simulink model "elastic_robot_arm_robust_controller"  (R2018b)
settings: Solver=ode8  StartTime=0.0  StopTime=50  FixedStep=0.001  RelTol=1e-3
undefined symbols (not defined in the file or in its folder): sigbuilder_block
settings Model: Creator=TUAN HUA  LastModifiedBy=Tuan Hua

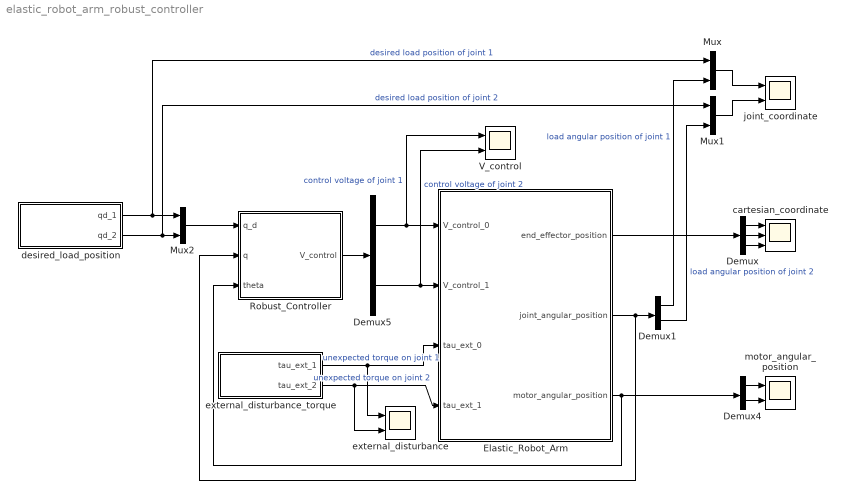
== system elastic_robot_arm_robust_controller ==
  Demux : Demux  Outputs=3
  Demux1 : Demux  Outputs=2
  Demux4 : Demux  Outputs=2
  Demux5 : Demux  Outputs=2
  Elastic_Robot_Arm : Subsystem  mask{ml0=6, Ilzz0=0.1, K0=1200.0, ml1=4, Ilzz1=0.1, K1=1440.0}
      mask prompts: ml0 "Link mass (kg) (defaut: 6)"; Ilzz0 "Link inertia (kg·m^2) (defaut: 0.1)"; K0 "Spring stiffness (N/m) (default: 1500)"; ml1 "Link mass (kg) (defaut: 4)"; Ilzz1 "Link inertia (kg·m^2) (defaut: 0.1)"; K1 "Spring stiffness (N/m) (default: 1200)"
      mask DialogControl Container1 Prompt: Joint 1
      mask DialogControl Container2 Prompt: Joint 2
      mask DialogControl Control1 Prompt: Reset to default
      mask DialogControl Control1 Callback:
      | robot_model = Simulink.Mask.get('elastic_robot_arm_robust_controller/Elastic_Robot_Arm');
      | 
      | % ml0
      | param = robot_model.Parameters(1);
      | param.set('Value', '6');
      | 
      | % Ilzz0
      | param = robot_model.Parameters(2);
      | param.set('Value', '0.1');
      | 
      | % K0
      | param = robot_model.Parameters(3);
      | param.set('Value', '1500');
      | 
      | % ml1
      | param = robot_model.Parameters(4);
      | param.set('Value', '4');
      | 
      | % Ilzz1
      | param = robot_model.Parameters(5);
      | param.set('Value', '0.1');
      | 
      | % K1
      | param = robot_model.Parameters(6);
      | param.set('Value', '1200');
  Mux : Mux  Inputs=2
  Mux1 : Mux  Inputs=2
  Mux2 : Mux  Inputs=2
  Robust_Controller : Subsystem
  V_control : Scope  NumInputPorts=2
  cartesian_coordinate : Scope  NumInputPorts=3
  desired_load_position : Subsystem  mask{inputType=Sine Waveform Input}
      mask prompts: inputType "Input Type"
      mask TypeOptions inputType: Sine Waveform Input | Square Waveform Input | Arbitrary Waveform Input
  external_disturbance : Scope  NumInputPorts=2
  external_disturbance_torque : Subsystem  mask{unexpectedTorqueType=No External Disturbance}
      mask prompts: unexpectedTorqueType "Unexpected Torque Type"
      mask TypeOptions unexpectedTorqueType: No External Disturbance | Unexpected Torque In Sine Waveform | Unexpected Torque In Pulse Form
  joint_coordinate : Scope  NumInputPorts=2
  motor_angular_position : Scope  NumInputPorts=2
  wires:
  Demux/3 -> cartesian_coordinate/3
  Demux/2 -> cartesian_coordinate/2
  Demux/1 -> cartesian_coordinate/1
  Elastic_Robot_Arm/1(end_effector_position) -> Demux/1
  Elastic_Robot_Arm/2(joint_angular_position) -> Robust_Controller/2(q), Demux1/1
  Elastic_Robot_Arm/3(motor_angular_position) -> Robust_Controller/3(theta), Demux4/1
  desired_load_position/1(qd_1) -> Mux/1, Mux2/1  "desired load position of joint 1"
  desired_load_position/2(qd_2) -> Mux1/1, Mux2/2  "desired load position of joint 2"
  Demux4/1 -> motor_angular_position/1
  Demux4/2 -> motor_angular_position/2
  Demux1/1 -> Mux/2  "load angular position of joint 1"
  Demux1/2 -> Mux1/2  "load angular position of joint 2"
  Mux/1 -> joint_coordinate/1
  Mux1/1 -> joint_coordinate/2
  Robust_Controller/1(V_control) -> Demux5/1
  Demux5/2 -> Elastic_Robot_Arm/2(V_control_1), V_control/2  "control voltage of joint 2"
  Demux5/1 -> Elastic_Robot_Arm/1(V_control_0), V_control/1  "control voltage of joint 1"
  Mux2/1 -> Robust_Controller/1(q_d)
  external_disturbance_torque/1(tau_ext_1) -> Elastic_Robot_Arm/3(tau_ext_0), external_disturbance/1  "unexpected torque on joint 1"
  external_disturbance_torque/2(tau_ext_2) -> Elastic_Robot_Arm/4(tau_ext_1), external_disturbance/2  "unexpected torque on joint 2"

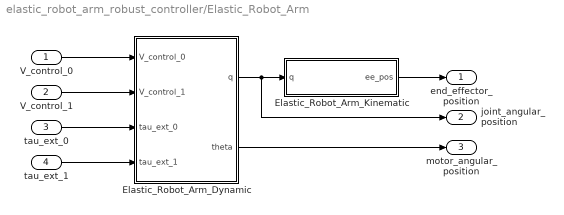
== system elastic_robot_arm_robust_controller/Elastic_Robot_Arm ==
  V_control_0 : Inport
  V_control_1 : Inport  Port=2
  tau_ext_0 : Inport  Port=3
  tau_ext_1 : Inport  Port=4
  Elastic_Robot_Arm_Dynamic : Subsystem
  Elastic_Robot_Arm_Kinematic : Subsystem
  end_effector_position : Outport
  joint_angular_position : Outport  Port=2
  motor_angular_position : Outport  Port=3
  wires:
  Elastic_Robot_Arm_Dynamic/2(theta) -> motor_angular_position/1
  Elastic_Robot_Arm_Kinematic/1(ee_pos) -> end_effector_position/1
  tau_ext_1/1 -> Elastic_Robot_Arm_Dynamic/4(tau_ext_1)
  tau_ext_0/1 -> Elastic_Robot_Arm_Dynamic/3(tau_ext_0)
  V_control_1/1 -> Elastic_Robot_Arm_Dynamic/2(V_control_1)
  V_control_0/1 -> Elastic_Robot_Arm_Dynamic/1(V_control_0)
  Elastic_Robot_Arm_Dynamic/1(q) -> Elastic_Robot_Arm_Kinematic/1(q), joint_angular_position/1

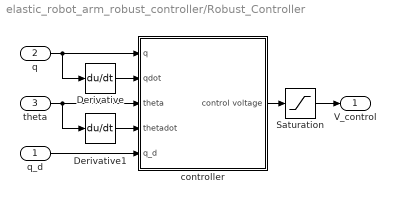
== system elastic_robot_arm_robust_controller/Robust_Controller ==
  q_d : Inport
  q : Inport  Port=2
  theta : Inport  Port=3
  Derivative : Derivative  CoefficientInTFapproximation=0
  Derivative1 : Derivative  CoefficientInTFapproximation=0
  Saturation : Saturate  UpperLimit=12  LowerLimit=-12
  controller : Subsystem
  V_control : Outport
  wires:
  q/1 -> controller/1(q), Derivative/1
  Derivative/1 -> controller/2(qdot)
  theta/1 -> Derivative1/1, controller/3(theta)
  Derivative1/1 -> controller/4(thetadot)
  q_d/1 -> controller/5(q_d)
  controller/1(control voltage) -> Saturation/1
  Saturation/1 -> V_control/1

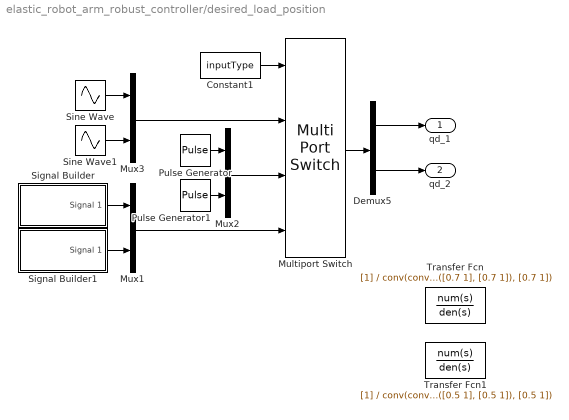
== system elastic_robot_arm_robust_controller/desired_load_position ==
  Constant1 : Constant  Value=inputType  OutDataTypeStr=uint8
  Demux5 : Demux  Outputs=2
  Multiport Switch : MultiPortSwitch
  Mux1 : Mux  Inputs=2
  Mux2 : Mux  Inputs=2
  Mux3 : Mux  Inputs=2
  Pulse Generator : DiscretePulseGenerator  PulseType=Time based  Period=20  PulseWidth=50
  Pulse Generator1 : DiscretePulseGenerator  PulseType=Time based  Period=20  PulseWidth=50
  Signal Builder : Subsystem  Tag=STV Subsys  LoadFcn=sigbuilder_block('load');  StartFcn=sigbuilder_block('start');  StopFcn=sigbuilder_block('stop');  ClipboardFcn=sigbuilder_block('clipboard');  mask(Sigbuilder block){tuvar=[0:10]}
      mask help: Simulink:masks:SigbuilderBlock_MD
      mask init:
      | if ~strcmp(get_param(bdroot(gcbh),'SimulationStatus'),'stopped') tuvar = sigbuilder_block('maskInit'); end
      settings: CopyFcn=sigbuilder_block('copy');  DeleteFcn=sigbuilder_block('delete');  ModelCloseFcn=sigbuilder_block('modelClose');  PreSaveFcn=sigbuilder_block('preSave');  PauseFcn=sigbuilder_block('pause');  ContinueFcn=sigbuilder_block('continue');  NameChangeFcn=sigbuilder_block('namechange');  OpenFcn=sigbuilder_block('open',[6 3 1012.5 474 ]);  CloseFcn=sigbuilder_block('close');
      mask Display: plot(0, 0, 100, 100,[2, 2, 32, 32, 2], [68, 8, 8, 68, 68],[32, 2], [38, 38], [32, 19, 2],[53, 60, 44], [32, 17, 17, 2],[16, 16, 31, 31]);txt = getActiveGroup(gcbh);text(2, 100, txt,'verticalAlignment', 'top');
  Signal Builder1 : Subsystem  Tag=STV Subsys  LoadFcn=sigbuilder_block('load');  StartFcn=sigbuilder_block('start');  StopFcn=sigbuilder_block('stop');  ClipboardFcn=sigbuilder_block('clipboard');  mask(Sigbuilder block){tuvar=[0:10]}
      mask help: Simulink:masks:SigbuilderBlock_MD
      mask init:
      | if ~strcmp(get_param(bdroot(gcbh),'SimulationStatus'),'stopped') tuvar = sigbuilder_block('maskInit'); end
      settings: CopyFcn=sigbuilder_block('copy');  DeleteFcn=sigbuilder_block('delete');  ModelCloseFcn=sigbuilder_block('modelClose');  PreSaveFcn=sigbuilder_block('preSave');  PauseFcn=sigbuilder_block('pause');  ContinueFcn=sigbuilder_block('continue');  NameChangeFcn=sigbuilder_block('namechange');  OpenFcn=sigbuilder_block('open',[6 0 1012.5 477.75 ]);  CloseFcn=sigbuilder_block('close');
      mask Display: plot(0, 0, 100, 100,[2, 2, 32, 32, 2], [68, 8, 8, 68, 68],[32, 2], [38, 38], [32, 19, 2],[53, 60, 44], [32, 17, 17, 2],[16, 16, 31, 31]);txt = getActiveGroup(gcbh);text(2, 100, txt,'verticalAlignment', 'top');
  Sine Wave : Sin  Frequency=0.25*pi  SampleTime=0
  Sine Wave1 : Sin  Frequency=0.25*pi  SampleTime=0
  Transfer Fcn : TransferFcn  Denominator=conv(conv([0.7 1], [0.7 1]), [0.7 1])
  Transfer Fcn1 : TransferFcn  Denominator=conv(conv([0.5 1], [0.5 1]), [0.5 1])
  qd_1 : Outport
  qd_2 : Outport  Port=2
  wires:
  Mux1/1 -> Multiport Switch/4
  Signal Builder1/1(Signal 1) -> Mux1/2
  Signal Builder/1(Signal 1) -> Mux1/1
  Demux5/2 -> qd_2/1
  Demux5/1 -> qd_1/1
  Constant1/1 -> Multiport Switch/1
  Sine Wave1/1 -> Mux3/2
  Mux2/1 -> Multiport Switch/3
  Pulse Generator/1 -> Mux2/1
  Pulse Generator1/1 -> Mux2/2
  Multiport Switch/1 -> Demux5/1
  Sine Wave/1 -> Mux3/1
  Mux3/1 -> Multiport Switch/2

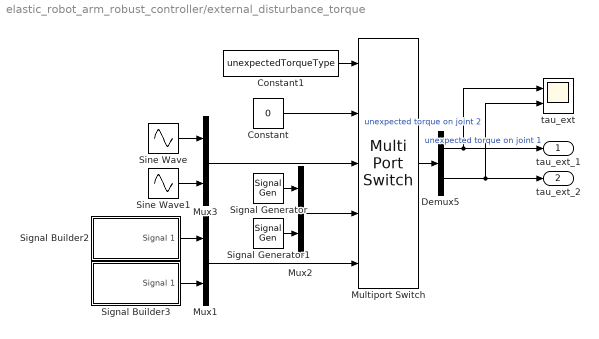
== system elastic_robot_arm_robust_controller/external_disturbance_torque ==
  Constant : Constant  Value=0
  Constant1 : Constant  Value=unexpectedTorqueType  OutDataTypeStr=uint8
  Demux5 : Demux  Outputs=2
  Multiport Switch : MultiPortSwitch  Inputs=4
  Mux1 : Mux  Inputs=2
  Mux2 : Mux  Inputs=2
  Mux3 : Mux  Inputs=2
  Signal Generator : SignalGenerator  WaveForm=square  Frequency=pi  Units=rad/sec
  Signal Generator1 : SignalGenerator  WaveForm=square  Frequency=0.5*pi  Units=rad/sec
  Signal Builder2 : Subsystem  Tag=STV Subsys  LoadFcn=sigbuilder_block('load');  StartFcn=sigbuilder_block('start');  StopFcn=sigbuilder_block('stop');  ClipboardFcn=sigbuilder_block('clipboard');  mask(Sigbuilder block){tuvar=[0:10]}
      mask help: Simulink:masks:SigbuilderBlock_MD
      mask init:
      | if ~strcmp(get_param(bdroot(gcbh),'SimulationStatus'),'stopped') tuvar = sigbuilder_block('maskInit'); end
      settings: CopyFcn=sigbuilder_block('copy');  DeleteFcn=sigbuilder_block('delete');  ModelCloseFcn=sigbuilder_block('modelClose');  PreSaveFcn=sigbuilder_block('preSave');  PauseFcn=sigbuilder_block('pause');  ContinueFcn=sigbuilder_block('continue');  NameChangeFcn=sigbuilder_block('namechange');  OpenFcn=sigbuilder_block('open',[0.75 27 1006.5 433.5 ]);  CloseFcn=sigbuilder_block('close');
      mask Display: plot(0, 0, 100, 100,[2, 2, 32, 32, 2], [68, 8, 8, 68, 68],[32, 2], [38, 38], [32, 19, 2],[53, 60, 44], [32, 17, 17, 2],[16, 16, 31, 31]);txt = getActiveGroup(gcbh);text(2, 100, txt,'verticalAlignment', 'top');
  Signal Builder3 : Subsystem  Tag=STV Subsys  LoadFcn=sigbuilder_block('load');  StartFcn=sigbuilder_block('start');  StopFcn=sigbuilder_block('stop');  ClipboardFcn=sigbuilder_block('clipboard');  mask(Sigbuilder block){tuvar=[0:10]}
      mask help: Simulink:masks:SigbuilderBlock_MD
      mask init:
      | if ~strcmp(get_param(bdroot(gcbh),'SimulationStatus'),'stopped') tuvar = sigbuilder_block('maskInit'); end
      settings: CopyFcn=sigbuilder_block('copy');  DeleteFcn=sigbuilder_block('delete');  ModelCloseFcn=sigbuilder_block('modelClose');  PreSaveFcn=sigbuilder_block('preSave');  PauseFcn=sigbuilder_block('pause');  ContinueFcn=sigbuilder_block('continue');  NameChangeFcn=sigbuilder_block('namechange');  OpenFcn=sigbuilder_block('open',[6 75 1012.5 437.25 ]);  CloseFcn=sigbuilder_block('close');
      mask Display: plot(0, 0, 100, 100,[2, 2, 32, 32, 2], [68, 8, 8, 68, 68],[32, 2], [38, 38], [32, 19, 2],[53, 60, 44], [32, 17, 17, 2],[16, 16, 31, 31]);txt = getActiveGroup(gcbh);text(2, 100, txt,'verticalAlignment', 'top');
  Sine Wave : Sin  Amplitude=5  Frequency=4*pi  SampleTime=0
  Sine Wave1 : Sin  Amplitude=5  Frequency=4*pi  SampleTime=0
  tau_ext : Scope  NumInputPorts=2
  tau_ext_1 : Outport
  tau_ext_2 : Outport  Port=2
  wires:
  Constant/1 -> Multiport Switch/2
  Mux3/1 -> Multiport Switch/3
  Sine Wave/1 -> Mux3/1
  Multiport Switch/1 -> Demux5/1
  Signal Generator1/1 -> Mux2/2
  Signal Generator/1 -> Mux2/1
  Mux2/1 -> Multiport Switch/4
  Sine Wave1/1 -> Mux3/2
  Constant1/1 -> Multiport Switch/1
  Demux5/1 -> tau_ext_1/1, tau_ext/1  "unexpected torque on joint 1"
  Demux5/2 -> tau_ext/2, tau_ext_2/1  "unexpected torque on joint 2"
  Signal Builder2/1(Signal 1) -> Mux1/1
  Signal Builder3/1(Signal 1) -> Mux1/2
  Mux1/1 -> Multiport Switch/5

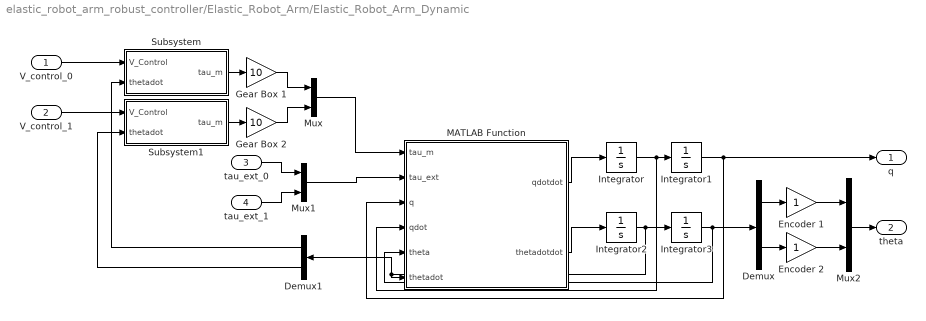
== system elastic_robot_arm_robust_controller/Elastic_Robot_Arm/Elastic_Robot_Arm_Dynamic ==
  V_control_0 : Inport
  V_control_1 : Inport  Port=2
  tau_ext_0 : Inport  Port=3
  tau_ext_1 : Inport  Port=4
  Demux : Demux  Outputs=2
  Demux1 : Demux  Outputs=2
  Encoder 1 : Gain
  Encoder 2 : Gain
  Gear Box 1 : Gain  Gain=10
  Gear Box 2 : Gain  Gain=10
  Integrator{,1..3} (4 alike) : Integrator  InitialCondition=[0;0]
  MATLAB Function : MATLAB Function  TreatAsAtomicUnit=on
  Mux : Mux  Inputs=2
  Mux1 : Mux  Inputs=2
  Mux2 : Mux  Inputs=2
  Subsystem : Subsystem
  Subsystem1 : Subsystem
  q : Outport
  theta : Outport  Port=2
  wires:
  Demux1/2 -> Subsystem1/2(thetadot)
  Demux1/1 -> Subsystem/2(thetadot)
  Subsystem1/1(tau_m) -> Gear Box 2/1
  Subsystem/1(tau_m) -> Gear Box 1/1
  Encoder 2/1 -> Mux2/2
  Gear Box 2/1 -> Mux/2
  Demux/2 -> Encoder 2/1
  V_control_1/1 -> Subsystem1/1(V_Control)
  Encoder 1/1 -> Mux2/1
  Demux/1 -> Encoder 1/1
  Mux2/1 -> theta/1
  Gear Box 1/1 -> Mux/1
  Mux/1 -> MATLAB Function/1(tau_m)
  Mux1/1 -> MATLAB Function/2(tau_ext)
  tau_ext_1/1 -> Mux1/2
  V_control_0/1 -> Subsystem/1(V_Control)
  tau_ext_0/1 -> Mux1/1
  Integrator3/1 -> Demux/1, MATLAB Function/5(theta)
  Integrator2/1 -> Demux1/1, MATLAB Function/6(thetadot), Integrator3/1
  MATLAB Function/2(thetadotdot) -> Integrator2/1
  Integrator1/1 -> q/1, MATLAB Function/3(q)
  Integrator/1 -> Integrator1/1, MATLAB Function/4(qdot)
  MATLAB Function/1(qdotdot) -> Integrator/1

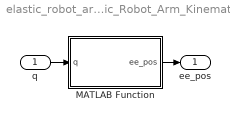
== system elastic_robot_arm_robust_controller/Elastic_Robot_Arm/Elastic_Robot_Arm_Kinematic ==
  q : Inport
  MATLAB Function : MATLAB Function  TreatAsAtomicUnit=on
  ee_pos : Outport
  wires:
  MATLAB Function/1(ee_pos) -> ee_pos/1
  q/1 -> MATLAB Function/1(q)

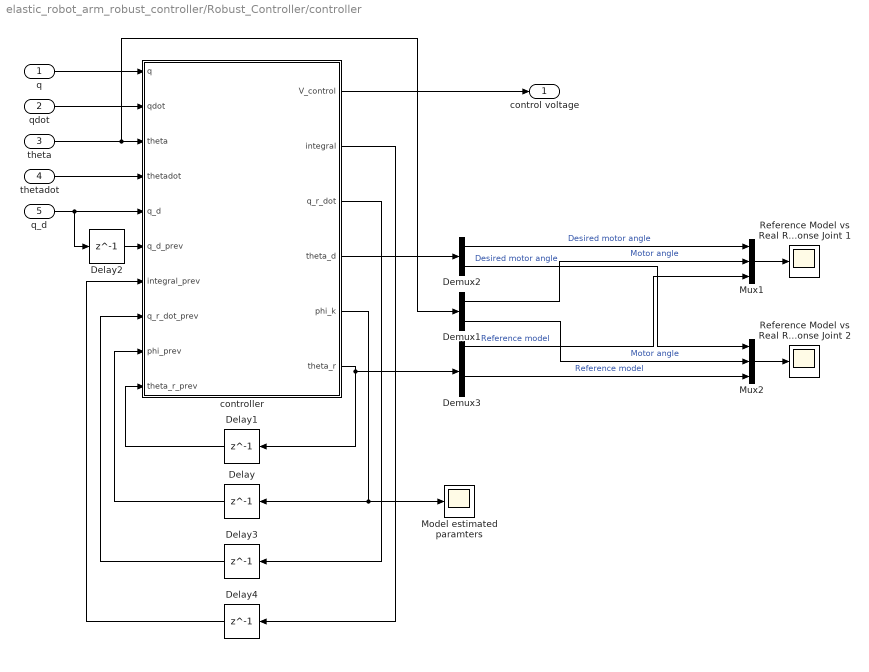
== system elastic_robot_arm_robust_controller/Robust_Controller/controller ==
  q : Inport
  qdot : Inport  Port=2
  theta : Inport  Port=3
  thetadot : Inport  Port=4
  q_d : Inport  Port=5
  Delay : Delay  DelayLength=1  InitialCondition=[5.9; 1.1; 3.1; 2.5; 0.9; 5.9; 1.1; 3.1; 2.5; 0.9]
  Delay1 : Delay  DelayLength=1  InitialCondition=[0; 0; 0; 0]
  Delay2 : Delay  DelayLength=1  InitialCondition=0
  Delay3 : Delay  DelayLength=1  InitialCondition=[0; 0]
  Delay4 : Delay  DelayLength=1  InitialCondition=[0; 0]
  Demux1 : Demux  Outputs=2
  Demux2 : Demux  Outputs=2
  Demux3 : Demux
  Model estimated paramters : Scope
  Mux1 : Mux  Inputs=3
  Mux2 : Mux  Inputs=3
  Reference Model vs Real Response Joint 1 : Scope
  Reference Model vs Real Response Joint 2 : Scope
  controller : MATLAB Function  TreatAsAtomicUnit=on
  control voltage : Outport
  wires:
  qdot/1 -> controller/2(qdot)
  theta/1 -> Demux1/1, controller/3(theta)
  thetadot/1 -> controller/4(thetadot)
  q/1 -> controller/1(q)
  controller/1(V_control) -> control voltage/1
  controller/6(theta_r) -> Delay1/1, Demux3/1
  controller/4(theta_d) -> Demux2/1
  Delay2/1 -> controller/6(q_d_prev)
  q_d/1 -> Delay2/1, controller/5(q_d)
  Delay/1 -> controller/9(phi_prev)
  Delay1/1 -> controller/10(theta_r_prev)
  controller/5(phi_k) -> Model estimated paramters/1, Delay/1
  controller/3(q_r_dot) -> Delay3/1
  Delay3/1 -> controller/8(q_r_dot_prev)
  controller/2(integral) -> Delay4/1
  Delay4/1 -> controller/7(integral_prev)
  Demux2/1 -> Mux1/1  "Desired motor angle"
  Demux1/1 -> Mux1/2  "Motor angle"
  Demux3/1 -> Mux1/3  "Reference model"
  Demux3/3 -> Mux2/3  "Reference model"
  Demux1/2 -> Mux2/2  "Motor angle"
  Demux2/2 -> Mux2/1  "Desired motor angle"
  Mux1/1 -> Reference Model vs Real Response Joint 1/1
  Mux2/1 -> Reference Model vs Real Response Joint 2/1

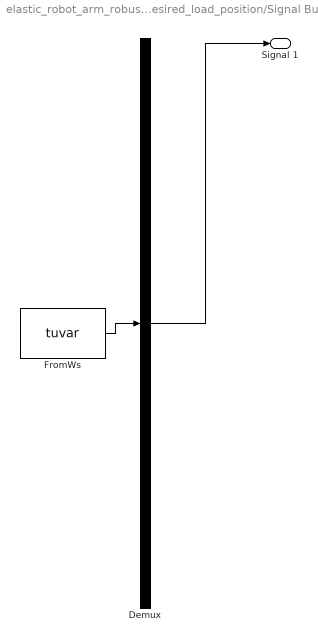
== system elastic_robot_arm_robust_controller/desired_load_position/Signal Builder ==
  Demux : Demux  Tag=STV Demux  Outputs=1
  FromWs : FromWorkspace  Tag=STV FromWs  VariableName=tuvar  SampleTime=0
      SigBuilderData=|
      | common.afterFinalStr = 'Extrapolate'
      | common.sampleTime = 0
      | dataSet.timeRange = [0 200]
      | dataSet.name = 'Group 1'
      | sbobj.Groups.Name = 'Group 1'
      | sbobj.Groups.Signals.Name = 'Signal 1'
      | sbobj.Groups.Signals.XData = [0 20 20 40 40 60 60 80 80 99.5 99.5 120 120 130 130 140 140 150 150 160 160 200]
      | sbobj.Groups.Signals.YData = [0.51 0.51 -0.49 -0.49 0.01 0.01 1.01 1.01 0.01 0.01 -0.49 -0.49 -0.99 -0.99 -0.49 -0.49 0.01 0.01 0.51 0.51 1 1]
      | sbobj.Groups.TimeRange = [0 200]
  Signal 1 : Outport  Tag=STV Outport
  wires:
  FromWs/1 -> Demux/1
  Demux/1 -> Signal 1/1

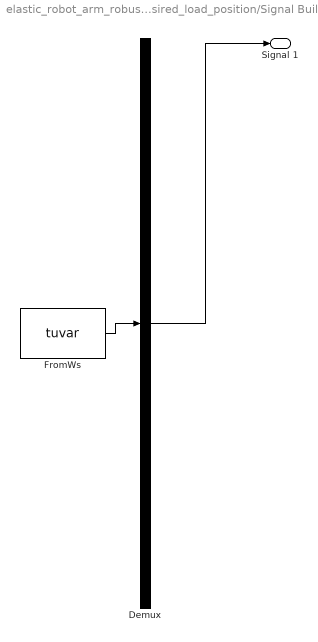
== system elastic_robot_arm_robust_controller/desired_load_position/Signal Builder1 ==
  Demux : Demux  Tag=STV Demux  Outputs=1
  FromWs : FromWorkspace  Tag=STV FromWs  VariableName=tuvar  SampleTime=0
      SigBuilderData=|
      | common.afterFinalStr = 'Extrapolate'
      | common.sampleTime = 0
      | dataSet.timeRange = [0 200]
      | dataSet.name = 'Group 1'
      | sbobj.Groups.Name = 'Group 1'
      | sbobj.Groups.Signals.Name = 'Signal 1'
      | sbobj.Groups.Signals.XData = [0 20 20 30 30 40 40 60 60 80 80 100 100 120 120 125 125 130 130 135 135 140 140 150 150 200]
      | sbobj.Groups.Signals.YData = [0.5 0.5 0 0 -0.2 -0.2 -0.4 -0.4 -0.5 -0.5 0 0 -1 -1 -0.5 -0.5 0 0 0.5 0.5 1 1 -0.5 -0.5 0.6 0.6]
      | sbobj.Groups.TimeRange = [0 200]
  Signal 1 : Outport  Tag=STV Outport
  wires:
  Demux/1 -> Signal 1/1
  FromWs/1 -> Demux/1

== system elastic_robot_arm_robust_controller/external_disturbance_torque/Signal Builder2 ==
  Demux : Demux  Tag=STV Demux  Outputs=1
  FromWs : FromWorkspace  Tag=STV FromWs  VariableName=tuvar  SampleTime=0
      SigBuilderData=|
      | common.afterFinalStr = 'Extrapolate'
      | common.sampleTime = 0
      | dataSet.timeRange = [0 200]
      | dataSet.name = 'Group 1'
      | sbobj.Groups.Name = 'Group 1'
      | sbobj.Groups.Signals.Name = 'Signal 1'
      | sbobj.Groups.Signals.XData = [0 20 20 40 40 80 80 120 120 200]
      | sbobj.Groups.Signals.YData = [0 0 -0.3 -0.3 0 0 0.4 0.4 0 0]
      | sbobj.Groups.TimeRange = [0 200]
  Signal 1 : Outport  Tag=STV Outport
  wires:
  FromWs/1 -> Demux/1
  Demux/1 -> Signal 1/1

== system elastic_robot_arm_robust_controller/external_disturbance_torque/Signal Builder3 ==
  Demux : Demux  Tag=STV Demux  Outputs=1
  FromWs : FromWorkspace  Tag=STV FromWs  VariableName=tuvar  SampleTime=0
      SigBuilderData=|
      | common.afterFinalStr = 'Extrapolate'
      | common.sampleTime = 0
      | dataSet.timeRange = [0 200]
      | dataSet.name = 'Group 1'
      | sbobj.Groups.Name = 'Group 1'
      | sbobj.Groups.Signals.Name = 'Signal 1'
      | sbobj.Groups.Signals.XData = [0 20 20 40 40 160 160 180 180 200]
      | sbobj.Groups.Signals.YData = [0 0 -0.3 -0.3 0 0 0.5 0.5 0 0]
      | sbobj.Groups.TimeRange = [0 200]
  Signal 1 : Outport  Tag=STV Outport
  wires:
  Demux/1 -> Signal 1/1
  FromWs/1 -> Demux/1

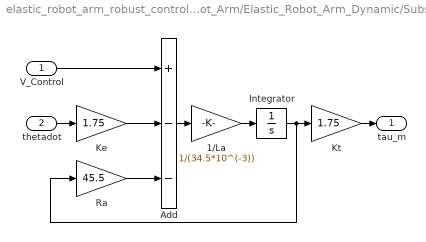
== system elastic_robot_arm_robust_controller/Elastic_Robot_Arm/Elastic_Robot_Arm_Dynamic/Subsystem ==
  V_Control : Inport
  thetadot : Inport  Port=2
  1/La : Gain  Gain=1/(34.5*10^(-3))
  Add : Sum  Inputs=+--
  Integrator : Integrator
  Ke : Gain  Gain=1.75
  Kt : Gain  Gain=1.75
  Ra : Gain  Gain=45.5
  tau_m : Outport
  wires:
  1/La/1 -> Integrator/1
  Add/1 -> 1/La/1
  Ra/1 -> Add/3
  Ke/1 -> Add/2
  V_Control/1 -> Add/1
  Integrator/1 -> Kt/1, Ra/1
  Kt/1 -> tau_m/1
  thetadot/1 -> Ke/1

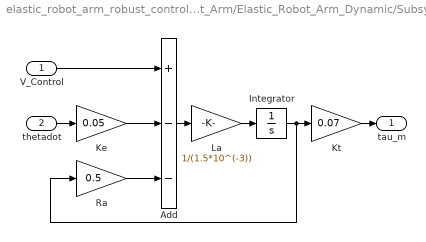
== system elastic_robot_arm_robust_controller/Elastic_Robot_Arm/Elastic_Robot_Arm_Dynamic/Subsystem1 ==
  V_Control : Inport
  thetadot : Inport  Port=2
  Add : Sum  Inputs=+--
  Integrator : Integrator
  Ke : Gain  Gain=0.05
  Kt : Gain  Gain=0.07
  La : Gain  Gain=1/(1.5*10^(-3))
  Ra : Gain  Gain=0.5
  tau_m : Outport
  wires:
  thetadot/1 -> Ke/1
  Kt/1 -> tau_m/1
  Integrator/1 -> Ra/1, Kt/1
  V_Control/1 -> Add/1
  Ke/1 -> Add/2
  Ra/1 -> Add/3
  Add/1 -> La/1
  La/1 -> Integrator/1

== matlab function elastic_robot_arm_robust_controller/Elastic_Robot_Arm/Elastic_Robot_Arm_Kinematic/MATLAB Function ==
  data: q input; ee_pos output
function ee_pos = kinematic(q)

    % Link length
    l0 = 0.1;
    l1 = 0.1;
    
    q_0 = q(1);
    q_1 = q(2);
    
    H2_0 = [[ cos(q_0)*cos(q_1), -sin(q_0), -cos(q_0)*sin(q_1), l1*cos(q_0)*cos(q_1)]
            [ cos(q_1)*sin(q_0),  cos(q_0), -sin(q_0)*sin(q_1), l1*cos(q_1)*sin(q_0)]
            [          sin(q_1),         0,           cos(q_1),     l0 + l1*sin(q_1)]
            [                 0,         0,                  0,                    1]];

    ee_pos = H2_0(1:3,4);

== matlab function elastic_robot_arm_robust_controller/Elastic_Robot_Arm/Elastic_Robot_Arm_Dynamic/MATLAB Function ==
  data: tau_m input; tau_ext input; q input; qdot input; theta input; qdotdot output; thetadotdot output; thetadot input; ml0 parameter; ml1 parameter; Ilzz0 parameter; Ilzz1 parameter; K0 parameter; K1 parameter
function [qdotdot, thetadotdot] = dynamic(tau_m, tau_ext, q, qdot, theta, thetadot, ml0, ml1, Ilzz0, Ilzz1, K0, K1)
    % Link length
    l0 = 0.3;
    l1 = 0.3;
    % Link and motor mass
%     ml0 = 6;
%     ml1 = 4;
    mm0 = 1;
    mm1 = 1;
    % Link and motor inertia
    Ilxx0 = 0;
    Ilyy0 = 0;
%     Ilzz0 = 0.1;
    Ilxx1 = 0;
    Ilyy1 = 0;
%     Ilzz1 = 0.1;
    Im0 = 0.003;
    Im1 = 0.003;
    % Link and motor damping coefficient
    Dm0 = 0.027;
    Dm1 = 0.027;
    Dl0 = 0.2;
    Dl1 = 0.2;
    % Gravitational constant
    g = 9.81;
    % String stiffness and damping coefficient
%     K0 = 1500;
%     K1 = 1200;
    % Gear ratio
    N0 = 10;
    N1 = 10;
    
    q0 = q(1);
    q1 = q(2);
    qdot0 = qdot(1);
    qdot1 = qdot(2);
    
    % Mass matrix
    M = [[ Ilzz0 + Ilzz1 + (l1^2*ml1)/4 - (l1^2*ml1*sin(q1)^2)/4,                                                        0]
         [                                                     0, Ilyy1 + (l1^2*ml1)/4 + Ilxx1*sin(q0)^2 - Ilyy1*sin(q0)^2]];
    
    % Centrifugal and Coriolis forces
    C = zeros(2,2);
    C(1,1) = -(l1^2*ml1*qdot1*sin(2*q1))/8;
    C(1,2) = -(qdot1*sin(2*q0)*(Ilxx1 - Ilyy1))/2;
    C(2,1) = (qdot1*sin(2*q0)*(Ilxx1 - Ilyy1))/2;
    C(2,2) = 0;
    
    % Gravitational forces
    G = zeros(2,1);
    G(1,1) = 0;
    G(2,1) = ml1*g*(l1/2)*cos(q1);

    % Dynamic equation in load side
    Dl = [Dl0,   0
            0, Dl1];
    K = [K0 0
         0  K1];
    tau_s = K*(theta - q);
    qdotdot = inv(M)*(tau_ext + tau_s - C*qdot - G - Dl*qdot);
    
    % Dynamic equation in motor side
    Dm = [Dm0,   0
            0, Dm1];
    B = [[Im0*(N0^2), 0]
         [         0, Im1*(N1^2)]];
    thetadotdot = inv(B)*(tau_m - tau_s - Dm*thetadot);

== matlab function elastic_robot_arm_robust_controller/Robust_Controller/controller/controller ==
  data: q input; qdot input; theta input; thetadot input; q_d input; q_d_prev input; integral_prev input; q_r_dot_prev input; V_control output; integral output; q_r_dot output; theta_d output; phi_prev input; theta_r_prev input; phi_k output; theta_r output
function [V_control, integral, q_r_dot, theta_d, phi_k, theta_r] = controller(q, qdot, theta, thetadot,...
                        q_d, q_d_prev, integral_prev, q_r_dot_prev, phi_prev, theta_r_prev)

    [theta_d, q_r_dot, integral] = robust_controller(q_d, q_d_prev, q, qdot, q_r_dot_prev, integral_prev);

    q0 = q(1);
    q1 = q(2);
    qdot0 = qdot(1);
    qdot1 = qdot(2);
    theta0 = theta(1);
    theta1 = theta(2);
    thetadot0 = thetadot(1);
    thetadot1 = thetadot(2);
    theta_d_0 = theta_d(1);
    theta_d_1 = theta_d(2);
    phi_prev_0 = phi_prev(1:5,1);
    phi_prev_1 = phi_prev(6:10,1);
    theta_r_prev_0 = theta_r_prev(1:2,1);
    theta_r_prev_1 = theta_r_prev(3:4,1);
    % Joint 0
    [V_control_0, phi_k_0, theta_r_0] = mrac(q0, qdot0, theta0, thetadot0,... 
                      theta_d_0, phi_prev_0, theta_r_prev_0);
    % Joint 1
    [V_control_1, phi_k_1, theta_r_1] = mrac(q1, qdot1, theta1, thetadot1,... 
                      theta_d_1, phi_prev_1, theta_r_prev_1);

    % Output data
    V_control = [V_control_0
                 V_control_1];
    phi_k = [phi_k_0
             phi_k_1];
    theta_r = [theta_r_0
               theta_r_1];
